simulink model "Roadsense_MotionPrediction"  (R2025b)
settings: Solver=FixedStepDiscrete  StartTime=0.0  StopTime=1.0  FixedStep=RsTsBase  RelTol=1e-3
undefined symbols (not defined in the file or in its folder): RsMaxPredictionModes, RsMaxTracks, RsPredictionSteps, RsTsPlanning
settings Model: DataDictionary=Roadsense_Data.sldd  Creator=ragur  LastModifiedBy=ragur

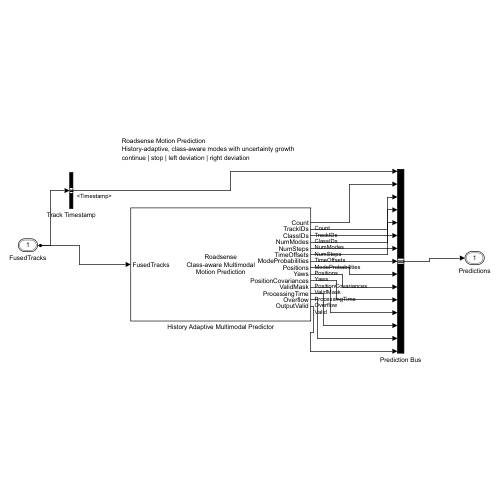
[thumbnail: Simulink's stored preview of the top-level diagram]
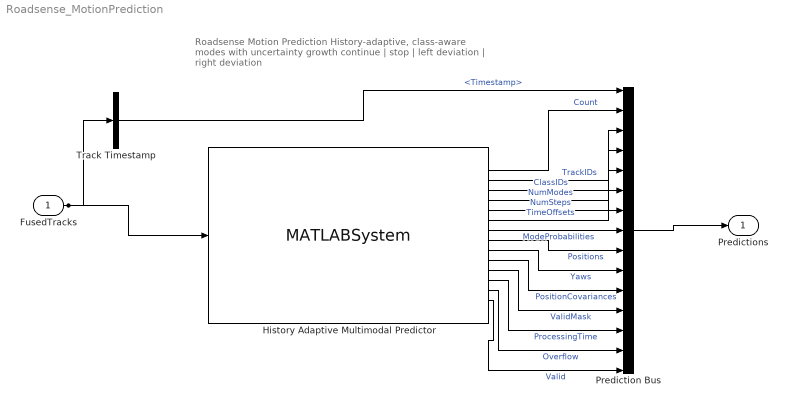
== system Roadsense_MotionPrediction ==
  note: Roadsense Motion Prediction
      | History-adaptive, class-aware modes with uncertainty growth
      | continue | stop | left deviation | right deviation
  FusedTracks : Inport  OutDataTypeStr=Bus: RsFusedTrackListBus  PortDimensions=1  SampleTime=RsTsPlanning
  History Adaptive Multimodal Predictor : MATLABSystem  System=RoadsenseMotionPredictionSystem  MaxTracks=double(RsMaxTracks)  MaxModes=double(RsMaxPredictionModes)  PredictionSteps=double(RsPredictionSteps)  PredictionStep=RsPredictionStep  HistoryGain=RsPredictionHistoryGain  VehicleTurnRate=RsPredictionVehicleTurnRate  VulnerableTurnRate=RsPredictionVulnerableTurnRate  VehicleBrake=RsPredictionVehicleBrake  VulnerableBrake=RsPredictionVulnerableBrake  MinimumModeProbability=RsPredictionMinimumModeProbability  SimulateUsing=Interpreted execution
      mask Type: RoadsenseMotionPredictionSystem
  Prediction Bus : BusCreator  Inputs=15  OutDataTypeStr=Bus: RsMotionPredictionListBus
  Track Timestamp : BusSelector  OutputSignals=Timestamp
  Predictions : Outport  OutDataTypeStr=Bus: RsMotionPredictionListBus
  wires:
  FusedTracks/1 -> Track Timestamp/1, History Adaptive Multimodal Predictor/1
  Track Timestamp/1 -> Prediction Bus/1  "<Timestamp>"
  History Adaptive Multimodal Predictor/1 -> Prediction Bus/2  "Count"
  History Adaptive Multimodal Predictor/2 -> Prediction Bus/3  "TrackIDs"
  History Adaptive Multimodal Predictor/3 -> Prediction Bus/4  "ClassIDs"
  History Adaptive Multimodal Predictor/4 -> Prediction Bus/5  "NumModes"
  History Adaptive Multimodal Predictor/5 -> Prediction Bus/6  "NumSteps"
  History Adaptive Multimodal Predictor/6 -> Prediction Bus/7  "TimeOffsets"
  History Adaptive Multimodal Predictor/7 -> Prediction Bus/8  "ModeProbabilities"
  History Adaptive Multimodal Predictor/8 -> Prediction Bus/9  "Positions"
  History Adaptive Multimodal Predictor/9 -> Prediction Bus/10  "Yaws"
  History Adaptive Multimodal Predictor/10 -> Prediction Bus/11  "PositionCovariances"
  History Adaptive Multimodal Predictor/11 -> Prediction Bus/12  "ValidMask"
  History Adaptive Multimodal Predictor/12 -> Prediction Bus/13  "ProcessingTime"
  History Adaptive Multimodal Predictor/13 -> Prediction Bus/14  "Overflow"
  History Adaptive Multimodal Predictor/14 -> Prediction Bus/15  "Valid"
  Prediction Bus/1 -> Predictions/1
